simulink model "HANcoder_E407_TTA_Controller_v2"  (R2018b)
settings: Solver=FixedStepDiscrete  StartTime=0.0  StopTime=1  FixedStep=0.01  RelTol=1e-3
PreLoadFcn:
  | librarySetup
  | eval([bdroot,'_startup']) %Calling [modelName]_startup.m
values from neighbouring files (symbols this model uses):
  basic_cycle_duration_bc0 = TM_Reset_Board   + COMP_duration    (= 212)    [HANcoder_E407_TTA_Controller_v3_startup.m]
  basic_cycle_duration_bc1 = TM_Reset_Var_bc1 + COMP_duration    (= 288)    [HANcoder_E407_TTA_Controller_v3_startup.m]
  comm_delay_estimation1 = round(comm_delay_measured1*hardware_granularity/frequency_IRQ)    [HANcoder_E407_TTA_Controller_v3_startup.m]
  comm_delay_estimation2 = round(comm_delay_measured2*hardware_granularity/frequency_IRQ)    [HANcoder_E407_TTA_Controller_v3_startup.m]
  COMM_Period = 40    [HANcoder_E407_TTA_Controller_v3_startup.m]
  COMM_Phase1 = Simulink.Parameter    [HANcoder_E407_TTA_Controller_v3_startup.m]
  COMM_Phase2 = Simulink.Parameter    [HANcoder_E407_TTA_Controller_v3_startup.m]
  COMP_duration = 4    [HANcoder_E407_TTA_Controller_v3_startup.m]
  Controller1_Board = 1    [HANcoder_E407_TTA_Controller_v3_startup.m]
  Controller2_Board = 2    [HANcoder_E407_TTA_Controller_v3_startup.m]
  Controller3_Board = 3    [HANcoder_E407_TTA_Controller_v3_startup.m]
  delta_max = 1    [HANcoder_E407_TTA_Controller_v3_startup.m]
  delta_min = -1    [HANcoder_E407_TTA_Controller_v3_startup.m]
  delta_precision = 6    [HANcoder_E407_TTA_Controller_v3_startup.m]
  e_width = 0.1    [HANcoder_E407_TTA_Controller_v3_startup.m]
  frequency_IRQ = 100    [HANcoder_E407_TTA_Controller_v3_startup.m]
  HANtuneOverride = Simulink.Parameter    [HANcoder_E407_TTA_Controller_v3_startup.m]
  hardware_granularity = 1000000    [HANcoder_E407_TTA_Controller_v3_startup.m]
  I_a = 2.25    [HANcoder_E407_TTA_Controller_v3_startup.m]
  I_f = 2.25    [HANcoder_E407_TTA_Controller_v3_startup.m]
  idle_time_init = basic_cycle_duration_bc0 + basic_cycle_duration_bc1    (= 500)    [HANcoder_E407_TTA_Controller_v3_startup.m]
  Input_Gen_Board = 4    [HANcoder_E407_TTA_Controller_v3_startup.m]
  LA_Clock_Gr = 1    [HANcoder_E407_TTA_Controller_v3_startup.m]
  LA_COMM_Err = 1    [HANcoder_E407_TTA_Controller_v3_startup.m]
  LA_MEX_Flag = 1    [HANcoder_E407_TTA_Controller_v3_startup.m]
  LA_Task_Act = 1    [HANcoder_E407_TTA_Controller_v3_startup.m]
  m_v = 100.0    (= 100)    [HANcoder_E407_TTA_Controller_v3_startup.m]
  Master_Role = 1    [HANcoder_E407_TTA_Controller_v3_startup.m]
  matrix_cycle_duration = basic_cycle_duration_bc0 + basic_cycle_duration_bc1    (= 500)    [HANcoder_E407_TTA_Controller_v3_startup.m]
  matrix_rows = 2    [HANcoder_E407_TTA_Controller_v3_startup.m]
  max_num_msgs_CAN1 = 2^Tx_bit_number-1    (= 7)    [HANcoder_E407_TTA_Controller_v3_startup.m]
  max_num_msgs_CAN2 = max_num_msgs_CAN1    (= 7)    [HANcoder_E407_TTA_Controller_v3_startup.m]
  OutControl1_ID = 23    [HANcoder_E407_TTA_Controller_v3_startup.m]
  OutControl2_ID = 24    [HANcoder_E407_TTA_Controller_v3_startup.m]
  OutEmulator_ID = 25    [HANcoder_E407_TTA_Controller_v3_startup.m]
  R_al = 0.10    (= 0.1)    [HANcoder_E407_TTA_Controller_v3_startup.m]
  R_ar = 0.10    (= 0.1)    [HANcoder_E407_TTA_Controller_v3_startup.m]
  R_fl = 0.10    (= 0.1)    [HANcoder_E407_TTA_Controller_v3_startup.m]
  R_fr = 0.10    (= 0.1)    [HANcoder_E407_TTA_Controller_v3_startup.m]
  SensorValues_ID = 22    [HANcoder_E407_TTA_Controller_v3_startup.m]
  SetValues_ID = 21    [HANcoder_E407_TTA_Controller_v3_startup.m]
  Slave_Role = 2    [HANcoder_E407_TTA_Controller_v3_startup.m]
  speed_k_d = Simulink.Parameter    [HANcoder_E407_TTA_Controller_v3_startup.m]
  speed_k_i = Simulink.Parameter    [HANcoder_E407_TTA_Controller_v3_startup.m]
  speed_k_p = Simulink.Parameter    [HANcoder_E407_TTA_Controller_v3_startup.m]
  speed_max = 10    [HANcoder_E407_TTA_Controller_v3_startup.m]
  speed_min = -10    [HANcoder_E407_TTA_Controller_v3_startup.m]
  speed_precision = 3    [HANcoder_E407_TTA_Controller_v3_startup.m]
  Sync_ID = 1    [HANcoder_E407_TTA_Controller_v3_startup.m]
  tau_max = 5    [HANcoder_E407_TTA_Controller_v3_startup.m]
  tau_min = -5    [HANcoder_E407_TTA_Controller_v3_startup.m]
  tau_range = abs(tau_max) + abs(tau_min)    [HANcoder_E407_TTA_Controller_v3_startup.m]
  theta_max = (speed_max/R_fr)*matrix_cycle_duration*frequency_IRQ/hardware_granularity    (= 5)    [HANcoder_E407_TTA_Controller_v3_startup.m]
  theta_min = (-1)*theta_max    (= -5)    [HANcoder_E407_TTA_Controller_v3_startup.m]
  theta_precision = 7-(fix(log2(theta_max))+1)    [HANcoder_E407_TTA_Controller_v3_startup.m]
  Tl_a = 0.6    [HANcoder_E407_TTA_Controller_v3_startup.m]
  Tl_f = 0.6    [HANcoder_E407_TTA_Controller_v3_startup.m]
  TM_Check_Output_Control1 = TM_COMM_Output_Control1 + COMM_duration    (= 188)    [HANcoder_E407_TTA_Controller_v3_startup.m]
  TM_Check_Output_Control2 = TM_COMM_Output_Control2 + COMM_duration    (= 232)    [HANcoder_E407_TTA_Controller_v3_startup.m]
  TM_Check_Output_Emulator = TM_COMM_Output_Emulator + COMM_duration    (= 280)    [HANcoder_E407_TTA_Controller_v3_startup.m]
  TM_Check_Sensor_Values = TM_COMM_Sensor_Values + COMM_duration    (= 132)    [HANcoder_E407_TTA_Controller_v3_startup.m]
  TM_Check_Set_Values = TM_COMM_Set_Values + COMM_duration    (= 88)    [HANcoder_E407_TTA_Controller_v3_startup.m]
  TM_Check_Sync = TM_COMM_Sync   + COMM_duration    (= 40)    [HANcoder_E407_TTA_Controller_v3_startup.m]
  TM_Check_TOuts = TM_Count_Vote3 + COMP_duration    (= 196)    [HANcoder_E407_TTA_Controller_v3_startup.m]
  TM_Check_Vote1 = TM_COMM_Vote1  + COMM_duration    (= 92)    [HANcoder_E407_TTA_Controller_v3_startup.m]
  TM_Check_Vote2 = TM_COMM_Vote2  + COMM_duration    (= 140)    [HANcoder_E407_TTA_Controller_v3_startup.m]
  TM_Check_Vote3 = TM_COMM_Vote3  + COMM_duration    (= 188)    [HANcoder_E407_TTA_Controller_v3_startup.m]
  TM_COMM_Output_Control1 = TM_Velocity + COMP_duration    (= 148)    [HANcoder_E407_TTA_Controller_v3_startup.m]
  TM_COMM_Output_Control2 = TM_Check_Output_Control1 + COMP_duration    (= 192)    [HANcoder_E407_TTA_Controller_v3_startup.m]
  TM_COMM_Output_Emulator = TM_TMR + COMP_duration    (= 240)    [HANcoder_E407_TTA_Controller_v3_startup.m]
  TM_COMM_Sensor_Values = TM_Check_Set_Values + COMP_duration    (= 92)    [HANcoder_E407_TTA_Controller_v3_startup.m]
  TM_COMM_Set_Values = TM_Update_LT + COMP_duration    (= 48)    [HANcoder_E407_TTA_Controller_v3_startup.m]
  TM_COMM_Sync = basic_cycle_start    (= 0)    [HANcoder_E407_TTA_Controller_v3_startup.m]
  TM_COMM_Vote1 = TM_Vote_Dec    + COMP_duration    (= 52)    [HANcoder_E407_TTA_Controller_v3_startup.m]
  TM_COMM_Vote2 = TM_Count_Vote1 + COMP_duration    (= 100)    [HANcoder_E407_TTA_Controller_v3_startup.m]
  TM_COMM_Vote3 = TM_Count_Vote2 + COMP_duration    (= 148)    [HANcoder_E407_TTA_Controller_v3_startup.m]
  TM_Count_Vote1 = TM_Check_Vote1 + COMP_duration    (= 96)    [HANcoder_E407_TTA_Controller_v3_startup.m]
  TM_Count_Vote2 = TM_Check_Vote2 + COMP_duration    (= 144)    [HANcoder_E407_TTA_Controller_v3_startup.m]
  TM_Count_Vote3 = TM_Check_Vote3 + COMP_duration    (= 192)    [HANcoder_E407_TTA_Controller_v3_startup.m]
  TM_Data_bc0 = TM_COMM_Sync    (= 0)    [HANcoder_E407_TTA_Controller_v3_startup.m]
  TM_Data_bc1 = TM_Data_bc0(1:4)    [HANcoder_E407_TTA_Controller_v3_startup.m]
  TM_New_Master = TM_Check_TOuts + COMP_duration    (= 200)    [HANcoder_E407_TTA_Controller_v3_startup.m]
  TM_Reset_Board = TM_Reset_Var   + COMP_duration    (= 208)    [HANcoder_E407_TTA_Controller_v3_startup.m]
  TM_Reset_Var = TM_New_Master  + COMP_duration    (= 204)    [HANcoder_E407_TTA_Controller_v3_startup.m]
  TM_Reset_Var_bc1 = TM_Check_Output_Emulator + COMP_duration    (= 284)    [HANcoder_E407_TTA_Controller_v3_startup.m]
  TM_Steer = TM_Check_Sensor_Values + COMP_duration    (= 136)    [HANcoder_E407_TTA_Controller_v3_startup.m]
  TM_TMR = TM_Check_Output_Control2 + COMP_duration    (= 236)    [HANcoder_E407_TTA_Controller_v3_startup.m]
  TM_Torque = TM_Steer + COMP_duration    (= 140)    [HANcoder_E407_TTA_Controller_v3_startup.m]
  TM_Type_bc0 = COMM    (= 0)    [HANcoder_E407_TTA_Controller_v3_startup.m]
  TM_Type_bc1 = TM_Type_bc0(1:4)    [HANcoder_E407_TTA_Controller_v3_startup.m]
  TM_Update_LT = TM_Check_Sync  + COMP_duration    (= 44)    [HANcoder_E407_TTA_Controller_v3_startup.m]
  TM_Velocity = TM_Torque + COMP_duration    (= 144)    [HANcoder_E407_TTA_Controller_v3_startup.m]
  TM_Vote_Dec = TM_Update_LT   + COMP_duration    (= 48)    [HANcoder_E407_TTA_Controller_v3_startup.m]
  torque_a_k_d = Simulink.Parameter    [HANcoder_E407_TTA_Controller_v3_startup.m]
  torque_a_k_i = Simulink.Parameter    [HANcoder_E407_TTA_Controller_v3_startup.m]
  torque_a_k_p = Simulink.Parameter    [HANcoder_E407_TTA_Controller_v3_startup.m]
  torque_f_k_d = Simulink.Parameter    [HANcoder_E407_TTA_Controller_v3_startup.m]
  torque_f_k_i = Simulink.Parameter    [HANcoder_E407_TTA_Controller_v3_startup.m]
  torque_f_k_p = Simulink.Parameter    [HANcoder_E407_TTA_Controller_v3_startup.m]
  torque_precision = 4    [HANcoder_E407_TTA_Controller_v3_startup.m]
  Vehicle_Em_Board = 5    [HANcoder_E407_TTA_Controller_v3_startup.m]
  Vote1_ID = 11    [HANcoder_E407_TTA_Controller_v3_startup.m]
  Vote2_ID = 12    [HANcoder_E407_TTA_Controller_v3_startup.m]
  Vote3_ID = 13    [HANcoder_E407_TTA_Controller_v3_startup.m]
undefined symbols (not defined in the file or in its folder): A0, A1, A2, A3, A4, CON2
libraries: hdlsllib x235, HANcoder_STM32_Target x25, simulink x3, simulink_extras x1
(part 2 of 22)

== system HANcoder_E407_TTA_Controller_v2/HANcoder STM32 Target - E407-STM32 algorithm/Global Ticks Increment/CAN2 Send ==
  note: Logic Analyzer - DEBUG
      | Message in transmission!
  note: Function call counter
  note: Log Activation CAN send
  note: DEBUG
  note: Logic Analyzer - DEBUG
  note: Transmission message count
      | Update
  Trigger : TriggerPort  TriggerType=function-call  VariantControl=Variant  PortDimensions=1
  Bus Selector : BusSelector  OutputSignals=Buffer_1,Buffer_2,Buffer_3,Buffer_4,Buffer_5,Buffer_6,Buffer_7,Buffer_8
  CAN send1 : Subsystem  Tag=HANcoder_TARGET_STM32_E407  AncestorBlock=HANcoder_STM32_Target/STM32-E407/CAN/CAN/CAN send  mask(CAN send){canBus=CAN 2, frameType=Standard (11 bit), inputNumber=8, dataType=uint8, byteOrder=off, tsamp=-1}
      mask prompts: canBus "CAN channel"; frameType "Identifier type"; inputNumber "Input ports"; dataType "Input datatype"; byteOrder "Byte order: Checked = MSB first, unchecked = LSB first."; tsamp "Sample time"
      mask help:
      | Function
      | ==========
      | Send a message on the CAN channel.
      |
      | Parameters
      | ==========
      | CAN channel:           The CAN channel to send the message on.
      | Identifier type:         normal or extended ID's
      | Input ports:              The amount of input ports
      | Input datatype:        The datatype of the input ports
      | Byte order:               Select MSB or LSB first
      | Sample time:            -1 or divisible by base sample time [seconds]
      |
      | Input
      | ==========
      | Port 1:                   CAN ID(uint32) in hexadecimal ie: hex2dec('0a')
      | Port 2..9                CAN message data
      mask init:
      | sfcn_can_send_mcb(canBus, frameType, inputNumber, dataType, byteOrder)
      settings: MoveFcn=drawLogos
      mask Help: web('sfcn_can_send.html');
      mask TypeOptions canBus: CAN 1 | CAN 2
      mask TypeOptions frameType: Standard (11 bit) | Extended (29 bit)
      mask TypeOptions dataType: int8 | uint8 | int16 | uint16 | int32 | uint32 | boolean
      mask Display:
      | fprintf('Send on\nCAN %x', canBus);
      | port_label('input', 1, 'ID');patch([140 146 146],[8 14 2],[1 0 0]);patch([148 148 154],[14 2 8],[0 0 0.35]);
  Cast To Double : DataTypeConversion  OutDataTypeStr=double
  Constant : Constant  OutDataTypeStr=boolean
  Constant3 : Constant  OutDataTypeStr=uint32
  Constant8 : Constant  Priority=2
  Data Store Memory1 : DataStoreMemory  DataStoreName=fcn_call_counter  ReadBeforeWriteMsg=warning  WriteAfterWriteMsg=warning  WriteAfterReadMsg=warning  ShowAdditionalParam=off  OutDataTypeStr=uint32
  Data Store Read : DataStoreRead  DataStoreName=fcn_call_counter
  Data Store Read1 : DataStoreRead  DataStoreName=Local_Ticks
  Data Store Read2 : DataStoreRead  DataStoreName=Msg_Tx_CAN2
  Data Store Read3 : DataStoreRead  DataStoreName=TxID_CAN2
  Data Store Read4 : DataStoreRead  Priority=1  DataStoreName=Tx_msg_count_CAN2
  Data Store Write : DataStoreWrite  DataStoreName=fcn_call_counter
  Data Store Write1 : DataStoreWrite  DataStoreName=Toggle_Pin_A0
  Data Store Write2 : DataStoreWrite  Priority=4  DataStoreName=Tx_msg_count_CAN2
  Data Type Conversion{,4..10} (8 alike) : DataTypeConversion  OutDataTypeStr=uint8
  Data Type Conversion1 : DataTypeConversion  OutDataTypeStr=uint32
  Get Free Running Counter1 : HANcoder_STM32_Target/STM32-E407/Timer Outputs/Get Free Running Counter  Tag=HANcoder_TARGET_STM32_E407  moduleID=TIM4 - CON PD - 15 & 16 &n/a & n/a  tsamp=-1
      settings: SourceProductName=HANcoder STM32 Target
  Plus : Sum  Priority=3
  Sum1 : Sum
  Terminator : Terminator
  Terminator4 : Terminator
  Terminator5 : Terminator
  wires:
  Constant/1 -> Data Store Write1/1
  Get Free Running Counter1/1 -> Terminator5/1  "FRC_Activation_CAN2_send"
  Data Store Read1/1 -> Terminator4/1  "Local_Ticks_Activation_CAN2_send"
  Sum1/1 -> Data Store Write/1  "TxCAN2_counter_s"
  Data Store Read/1 -> Sum1/2
  Constant3/1 -> Sum1/1
  Data Type Conversion7/1 -> CAN send1/6(In6)
  Data Type Conversion6/1 -> CAN send1/5(In5)
  Data Type Conversion4/1 -> CAN send1/3(In3)
  Data Type Conversion5/1 -> CAN send1/4(In4)
  Data Type Conversion8/1 -> CAN send1/7(In7)
  Data Type Conversion9/1 -> CAN send1/8(In8)
  Data Type Conversion1/1 -> CAN send1/1(In1)
  Data Type Conversion/1 -> CAN send1/2(In2)
  Data Type Conversion10/1 -> CAN send1/9(In9)
  Data Store Read3/1 -> Data Type Conversion1/1  "TxID_CAN2_s"
  Bus Selector/3 -> Data Type Conversion5/1  "<Buffer_3>"
  Bus Selector/2 -> Data Type Conversion4/1  "<Buffer_2>"
  Bus Selector/6 -> Data Type Conversion8/1  "<Buffer_6>"
  Bus Selector/4 -> Data Type Conversion6/1  "<Buffer_4>"
  Bus Selector/8 -> Data Type Conversion10/1  "<Buffer_8>"
  Data Store Read2/1 -> Bus Selector/1
  Bus Selector/7 -> Data Type Conversion9/1  "<Buffer_7>"
  Bus Selector/5 -> Data Type Conversion7/1  "<Buffer_5>"
  Data Store Read4/1 -> Plus/1
  Plus/1 -> Data Store Write2/1
  Constant8/1 -> Plus/2
  Bus Selector/1 -> Cast To Double/1, Data Type Conversion/1  "<Buffer_1>"
  Cast To Double/1 -> Terminator/1  "Tx_temporal_msg_CAN2"

== system HANcoder_E407_TTA_Controller_v2/HANcoder STM32 Target - E407-STM32 algorithm/Global Ticks Increment/If Action Subsystem ==
  note: CAN ID Init
  Action Port : ActionPort  ActionType=then
  Add : Sum  Inputs=++++
  Constant : Constant
  Constant1 : Constant  Value=2
  Constant2 : Constant  Value=4
  Constant3 : Constant  Value=8
  Digital Input4 : HANcoder_STM32_Target/STM32-E407/Digital Inputs/Digital Input  Tag=HANcoder_TARGET_STM32_E407  pinID=CON3 - D2 - 5V Tolerant  config=Pulldown  tsamp=-1
      settings: SourceProductName=HANcoder STM32 Target
  Digital Input5 : HANcoder_STM32_Target/STM32-E407/Digital Inputs/Digital Input  Tag=HANcoder_TARGET_STM32_E407  pinID=CON3 - D3 - 5V Tolerant  config=Pulldown  tsamp=-1
      settings: SourceProductName=HANcoder STM32 Target
  Digital Input6 : HANcoder_STM32_Target/STM32-E407/Digital Inputs/Digital Input  Tag=HANcoder_TARGET_STM32_E407  pinID=CON3 - D4 - 5V Tolerant  config=Pulldown  tsamp=-1
      settings: SourceProductName=HANcoder STM32 Target
  Digital Input7 : HANcoder_STM32_Target/STM32-E407/Digital Inputs/Digital Input  Tag=HANcoder_TARGET_STM32_E407  pinID=CON3 - D5 - 5V Tolerant  config=Pulldown  tsamp=-1
      settings: SourceProductName=HANcoder STM32 Target
  Multiply{,1..3} (4 alike) : Product
  Out1 : Outport
  wires:
  Constant1/1 -> Multiply1/1
  Add/1 -> Out1/1
  Constant3/1 -> Multiply3/1
  Constant2/1 -> Multiply2/1
  Multiply2/1 -> Add/3
  Digital Input7/1 -> Multiply3/2
  Digital Input5/1 -> Multiply1/2
  Multiply3/1 -> Add/4
  Multiply1/1 -> Add/2
  Digital Input6/1 -> Multiply2/2
  Multiply/1 -> Add/1
  Digital Input4/1 -> Multiply/2
  Constant/1 -> Multiply/1

== system HANcoder_E407_TTA_Controller_v2/HANcoder STM32 Target - E407-STM32 algorithm/Global Ticks Increment/Initialize Clock Schedule ==
  Enable : EnablePort
  Constant : Constant  OutDataTypeStr=uint16
  Constant1 : Constant  Value=3  OutDataTypeStr=uint8
  Constant2 : Constant
  Data Store Write : DataStoreWrite  DataStoreName=init_clock
  Schedule Compare Event : HANcoder_STM32_Target/STM32-E407/Timer Outputs/Schedule Compare Event  Tag=HANcoder_TARGET_STM32_E407  pin=TIM4 - CON PD - 15 - 5V Tolerant  tsamp=-1
      settings: SourceProductName=HANcoder STM32 Target
  wires:
  Constant/1 -> Schedule Compare Event/1
  Constant1/1 -> Schedule Compare Event/2
  Constant2/1 -> Data Store Write/1

== system HANcoder_E407_TTA_Controller_v2/HANcoder STM32 Target - E407-STM32 algorithm/Global Ticks Increment/Local Time generation ==
  note: Reschedule IRQ activation
  Clock_State : Inport
  function : TriggerPort  TriggerType=function-call  VariantControl=Variant
  Chart : Stateflow chart  TreatAsAtomicUnit=on
  Constant : Constant  Value=frequency_IRQ  OutDataTypeStr=uint16
  Constant1 : Constant  Value=3  OutDataTypeStr=uint8
  Constant2 : Constant  OutDataTypeStr=uint16
  Data Store Read : DataStoreRead  DataStoreName=Local_Ticks
  Data Store Read1 : DataStoreRead  DataStoreName=Local_Ticks
  Data Store Write : DataStoreWrite  DataStoreName=Local_Ticks
  Get Last Event Counter : HANcoder_STM32_Target/STM32-E407/Timer Outputs/Get Last Event Counter  Tag=HANcoder_TARGET_STM32_E407  pin=TIM4 - CON PD - 15 - 5V Tolerant  tsamp=-1
      settings: SourceProductName=HANcoder STM32 Target
  Schedule Compare Event1 : HANcoder_STM32_Target/STM32-E407/Timer Outputs/Schedule Compare Event  Tag=HANcoder_TARGET_STM32_E407  pin=TIM4 - CON PD - 15 - 5V Tolerant  tsamp=-1
      settings: SourceProductName=HANcoder STM32 Target
  Sum : Sum
  Sum1 : Sum
  Switch : Switch  Criteria=u2 > Threshold
  activate_CAN_management : Outport
  wires:
  Get Last Event Counter/1 -> Sum/1
  Constant/1 -> Sum/2
  Sum/1 -> Schedule Compare Event1/1
  Constant1/1 -> Schedule Compare Event1/2
  Data Store Read1/1 -> Switch/3
  Data Store Read/1 -> Sum1/1
  Constant2/1 -> Sum1/2
  Clock_State/1 -> Chart/1(Condition), Switch/2
  Switch/1 -> Data Store Write/1  "local_ticks_interrupt"
  Sum1/1 -> Switch/1
  Chart/1(Trigger_Signal()) -> activate_CAN_management/1

== system HANcoder_E407_TTA_Controller_v2/HANcoder STM32 Target - E407-STM32 algorithm/Global Ticks Increment/Measure EXecution time ==
  note: Measured Execution Time
  Trigger : TriggerPort  TriggerType=function-call  VariantControl=Variant
  Constant1 : Constant  Priority=1  Value=LA_MEX_Flag
  DEBUG - Toggle digital pin A3 : Subsystem  Priority=3
  Data Store Memory4 : DataStoreMemory  DataStoreName=A3_Pin_State  ReadBeforeWriteMsg=warning  WriteAfterWriteMsg=warning  WriteAfterReadMsg=warning  ShowAdditionalParam=off  OutDataTypeStr=boolean
  wires:
  Constant1/1 -> DEBUG - Toggle digital pin A3/Enable

== system HANcoder_E407_TTA_Controller_v2/HANcoder STM32 Target - E407-STM32 algorithm/Global Ticks Increment/Output Compare Init ==
  S-Function : S-Function  FunctionName=sfcn_timeout_init  SFunctionDeploymentMode=off  EnableBusSupport=off
  Term1 : Terminator
  wires:
  S-Function/1 -> Term1/1

== system HANcoder_E407_TTA_Controller_v2/HANcoder STM32 Target - E407-STM32 algorithm/Operation Mode/Flip Flop T ==
  T : Inport  OutDataTypeStr=boolean
  Clk : Inport  Port=2  OutDataTypeStr=boolean
  J-K Flip-Flop : simulink_extras/Flip Flops/J-K Flip-Flop  initial_condition=0
      settings: SourceProductName=Simulink
  Terminator : Terminator
  Q : Outport  OutDataTypeStr=boolean
  wires:
  J-K Flip-Flop/2 -> Terminator/1
  T/1 -> J-K Flip-Flop/3, J-K Flip-Flop/1
  J-K Flip-Flop/1 -> Q/1
  Clk/1 -> J-K Flip-Flop/2

== system HANcoder_E407_TTA_Controller_v2/HANcoder STM32 Target - E407-STM32 algorithm/Global Ticks Increment/CAN Management/Basic Cycle Increment ==
  note: Local Time Reset
  note: Basic cycle counter
  Enable : EnablePort
  Add : Sum
  Add1 : Sum  Inputs=+-
  Cast : DataTypeConversion  OutDataTypeStr=uint8
  Constant : Constant  Value=matrix_rows
  Data Store Read4 : DataStoreRead  DataStoreName=basic_cycle_count
  Data Store Read5 : DataStoreRead  DataStoreName=basic_cycle_count
  Data Store Write : DataStoreWrite  DataStoreName=Local_Ticks
  Data Store Write3 : DataStoreWrite  DataStoreName=basic_cycle_count
  Decrement : Constant  OutDataTypeStr=uint8
  Increment : Constant  OutDataTypeStr=uint8
  LessThanOrEqual : RelationalOperator  Operator=<  OutDataTypeStr=boolean  RndMeth=Simplest
  Reset : Constant  Value=0  OutDataTypeStr=uint16
  Switch : Switch  Criteria=u2 > Threshold
  wires:
  Switch/1 -> Data Store Write3/1  "bacic_cycle_s"
  Data Store Read5/1 -> LessThanOrEqual/1
  Add/1 -> Switch/1
  Increment/1 -> Add/2
  Data Store Read4/1 -> Add/1
  LessThanOrEqual/1 -> Switch/2
  Constant/1 -> Add1/1
  Reset/1 -> Cast/1, Data Store Write/1
  Decrement/1 -> Add1/2
  Add1/1 -> LessThanOrEqual/2
  Cast/1 -> Switch/3

== system HANcoder_E407_TTA_Controller_v2/HANcoder STM32 Target - E407-STM32 algorithm/Global Ticks Increment/CAN Management/DEBUG - Toggle digital pin A0 ==
  note: Change pin state
  note: Reset condition
  note: Toggle pin data stored
  Enable : EnablePort
  Constant : Constant  OutDataTypeStr=boolean
  Constant1 : Constant  Value=0  OutDataTypeStr=boolean
  Constant2 : Constant  Value=0  OutDataTypeStr=boolean
  Data Store Read : DataStoreRead  DataStoreName=A0_Pin_State
  Data Store Read1 : DataStoreRead  DataStoreName=A0_Pin_State
  Data Store Write : DataStoreWrite  DataStoreName=Toggle_Pin_A0
  Data Store Write1 : DataStoreWrite  DataStoreName=A0_Pin_State
  Digital Output : HANcoder_STM32_Target/STM32-E407/Digital Outputs/Digital Output  Tag=HANcoder_TARGET_STM32_E407  pinID=CON2 - A0  config=Open drain  tsamp=-1
      settings: SourceProductName=HANcoder STM32 Target
  Switch : Switch  Criteria=u2 > Threshold
  wires:
  Switch/1 -> Data Store Write1/1
  Data Store Read/1 -> Switch/2
  Constant/1 -> Switch/3
  Constant1/1 -> Switch/1
  Constant2/1 -> Data Store Write/1
  Data Store Read1/1 -> Digital Output/1

== system HANcoder_E407_TTA_Controller_v2/HANcoder STM32 Target - E407-STM32 algorithm/Global Ticks Increment/CAN Management/DEBUG - Toggle digital pin A1 ==
  note: Toggle pin data stored
  note: Reset condition
  note: Change pin state
  Enable : EnablePort
  Constant : Constant  OutDataTypeStr=boolean
  Constant1 : Constant  Value=0  OutDataTypeStr=boolean
  Constant2 : Constant  Value=0  OutDataTypeStr=boolean
  Data Store Read : DataStoreRead  DataStoreName=A1_Pin_State
  Data Store Read1 : DataStoreRead  DataStoreName=A1_Pin_State
  Data Store Write : DataStoreWrite  DataStoreName=Toggle_Pin_A1
  Data Store Write1 : DataStoreWrite  DataStoreName=A1_Pin_State
  Digital Output : HANcoder_STM32_Target/STM32-E407/Digital Outputs/Digital Output  Tag=HANcoder_TARGET_STM32_E407  pinID=CON2 - A1  config=Open drain  tsamp=-1
      settings: SourceProductName=HANcoder STM32 Target
  Switch : Switch  Criteria=u2 > Threshold
  wires:
  Data Store Read1/1 -> Digital Output/1
  Constant2/1 -> Data Store Write/1
  Constant1/1 -> Switch/1
  Constant/1 -> Switch/3
  Data Store Read/1 -> Switch/2
  Switch/1 -> Data Store Write1/1

== system HANcoder_E407_TTA_Controller_v2/HANcoder STM32 Target - E407-STM32 algorithm/Global Ticks Increment/CAN Management/DEBUG - Toggle digital pin A2 ==
  note: Toggle pin data stored
  note: Change pin state
  Enable : EnablePort
  Constant : Constant  OutDataTypeStr=boolean
  Constant1 : Constant  Value=0  OutDataTypeStr=boolean
  Data Store Read : DataStoreRead  DataStoreName=A2_Pin_State
  Data Store Read1 : DataStoreRead  DataStoreName=A2_Pin_State
  Data Store Write1 : DataStoreWrite  DataStoreName=A2_Pin_State
  Digital Output : HANcoder_STM32_Target/STM32-E407/Digital Outputs/Digital Output  Tag=HANcoder_TARGET_STM32_E407  pinID=CON2 - A2  config=Open drain  tsamp=-1
      settings: SourceProductName=HANcoder STM32 Target
  Switch : Switch  Criteria=u2 > Threshold
  wires:
  Data Store Read1/1 -> Digital Output/1
  Constant1/1 -> Switch/1
  Constant/1 -> Switch/3
  Data Store Read/1 -> Switch/2
  Switch/1 -> Data Store Write1/1

== system HANcoder_E407_TTA_Controller_v2/HANcoder STM32 Target - E407-STM32 algorithm/Global Ticks Increment/CAN Management/DEBUG - Toggle digital pin A4 ==
  note: Toggle pin data stored
  note: Change pin state
  Enable : EnablePort
  Constant : Constant  OutDataTypeStr=boolean
  Constant1 : Constant  Value=0  OutDataTypeStr=boolean
  Data Store Read : DataStoreRead  DataStoreName=A4_Pin_State
  Data Store Read1 : DataStoreRead  DataStoreName=A4_Pin_State
  Data Store Write1 : DataStoreWrite  DataStoreName=A4_Pin_State
  Digital Output : HANcoder_STM32_Target/STM32-E407/Digital Outputs/Digital Output  Tag=HANcoder_TARGET_STM32_E407  pinID=CON2 - A4  config=Open drain  tsamp=-1
      settings: SourceProductName=HANcoder STM32 Target
  Switch : Switch  Criteria=u2 > Threshold
  wires:
  Data Store Read1/1 -> Digital Output/1
  Constant1/1 -> Switch/1
  Constant/1 -> Switch/3
  Data Store Read/1 -> Switch/2
  Switch/1 -> Data Store Write1/1

== system HANcoder_E407_TTA_Controller_v2/HANcoder STM32 Target - E407-STM32 algorithm/Global Ticks Increment/CAN Management/Initialization ==
  Enable : EnablePort  PropagateVarSize=During execution
  AND : Logic  IconShape=distinctive  AllPortsSameDT=off  OutDataTypeStr=boolean
  Board nr1 : Constant
  Constant : Constant  Value=idle_time_init
  Data Store Memory : DataStoreMemory  DataStoreName=Initialization_Timeout  ReadBeforeWriteMsg=warning  WriteAfterWriteMsg=warning  WriteAfterReadMsg=warning  ShowAdditionalParam=off  OutDataTypeStr=boolean
  Data Store Memory1 : DataStoreMemory  DataStoreName=Delay_Counter  ReadBeforeWriteMsg=warning  WriteAfterWriteMsg=warning  WriteAfterReadMsg=warning  ShowAdditionalParam=off  OutDataTypeStr=double
  Data Store Read : DataStoreRead  DataStoreName=New_Msg_Ready_CAN1
  Data Store Read1 : DataStoreRead  DataStoreName=Initialization_Timeout
  Data Store Read2 : DataStoreRead  DataStoreName=New_Msg_Ready_CAN2
  Data Store Read4 : DataStoreRead  DataStoreName=Board_ID
  Data Store Write : DataStoreWrite  DataStoreName=Initialization_Timeout
  Data Store Write1 : DataStoreWrite  DataStoreName=Initialization_flag
  Delay : Subsystem
  Equal : RelationalOperator  Operator===  OutDataTypeStr=boolean  RndMeth=Simplest
  NOT : Logic  Operator=NOT  IconShape=distinctive  AllPortsSameDT=off  OutDataTypeStr=boolean
  OR : Logic  Operator=OR  IconShape=distinctive  AllPortsSameDT=off  OutDataTypeStr=boolean
  OR1 : Logic  Operator=OR  IconShape=distinctive  AllPortsSameDT=off  OutDataTypeStr=boolean
  RoleID and Global Time init : Subsystem  TreatAsAtomicUnit=on
  wires:
  Delay/1(Output) -> Data Store Write/1
  Constant/1 -> Delay/1(Input)
  NOT/1 -> Data Store Write1/1
  RoleID and Global Time init/1(Finish Initialization) -> NOT/1
  OR/1 -> RoleID and Global Time init/Enable
  Data Store Read1/1 -> AND/2, RoleID and Global Time init/1(Timeout Initialization)
  OR1/1 -> OR/2, RoleID and Global Time init/2(Reference message received)
  Data Store Read4/1 -> Equal/1
  Board nr1/1 -> Equal/2
  Equal/1 -> AND/1
  AND/1 -> OR/1
  Data Store Read/1 -> OR1/1
  Data Store Read2/1 -> OR1/2

== system HANcoder_E407_TTA_Controller_v2/HANcoder STM32 Target - E407-STM32 algorithm/Global Ticks Increment/CAN Management/LT_Update Desync_Positive ==
  note: Local Time Update with Positive Desync
      | This subsystem is only activated if we have to update
      | the local time with a positive desync. This is activated
      | at the end of the current Computational Task, so the
      | Local Time is updated until the tick before the next
      | Computational Task in the basic cycle. This way we
      | avoid missing tasks, as would happened when updating
      | the Local Time too quickly into the future.
  note: WARNING
      | TM_Type is currently defined as
      | COMM type 0
      | COMP type 1
  note: Constants bc0
  note: constants are defined in the _startup file
  note: Constants bc1
  Local Time : Inport
  Bacic_Cycle : Inport  Port=2
  Enable : EnablePort  PropagateVarSize=During execution
  Bus Selector : BusSelector  OutputSignals=signal1,signal2
  Bus Creator : BusCreator  Inputs=2
  Bus Creator1 : BusCreator  Inputs=2
  Constant : Constant  Value=TM_Data_bc0
  Constant1 : Constant  Value=TM_Type_bc0
  Constant2 : Constant  Value=COMM_Phase1
  Constant3 : Constant  Value=COMM_Phase2
  Constant4 : Constant  Value=TM_Data_bc1
  Constant5 : Constant  Value=TM_Type_bc1
  Constant8 : Constant  Value=0
  Equal : RelationalOperator  Operator===  OutDataTypeStr=boolean  RndMeth=Simplest
  Local Time Update with Positive Desync : Subsystem  TreatAsAtomicUnit=on
  MATLAB Function : MATLAB Function  TreatAsAtomicUnit=on
  Switch : Switch  Criteria=u2 > Threshold  AllowDiffInputSizes=on
  wires:
  MATLAB Function/1(result_time) -> Local Time Update with Positive Desync/1(Ticks until next COMP)
  Local Time/1 -> MATLAB Function/1(local_time)
  Constant8/1 -> Equal/2
  Bacic_Cycle/1 -> Equal/1
  Equal/1 -> Switch/2
  Constant/1 -> Bus Creator/1
  Constant1/1 -> Bus Creator/2
  Bus Creator/1 -> Switch/1
  Constant4/1 -> Bus Creator1/1
  Constant5/1 -> Bus Creator1/2
  Bus Creator1/1 -> Switch/3
  Switch/1 -> Bus Selector/1
  Bus Selector/1 -> MATLAB Function/2(TM_data)  "<signal1>"
  Bus Selector/2 -> MATLAB Function/3(TM_type)  "<signal2>"
  Constant3/1 -> MATLAB Function/5(phase2)
  Constant2/1 -> MATLAB Function/4(phase1)

== system HANcoder_E407_TTA_Controller_v2/HANcoder STM32 Target - E407-STM32 algorithm/Global Ticks Increment/CAN Management/Matrix Cycle Manager ==
  note: Controller boards condition
  note: Output Send_Message
      | Send: 1
      | Do not send: 0
  note: Output Receive_Message
      | Receive: 1
      | Do not receive: 0
  note: Output Receive_Message
      | Receive: 1
      | Do not receive: 0
  note: Output Send_Message
      | Send: 1
      | Do not send: 0
  Enable : EnablePort  PropagateVarSize=During execution
  Bus Selector : BusSelector  OutputSignals=signal1,signal2,signal3,signal4
  Bus Creator : BusCreator  Inputs=4
  Constant : Constant  Value=Controller1_Board
  Constant1 : Constant  Value=Controller2_Board
  Constant2 : Constant  Value=Controller3_Board
  Data Store Read : DataStoreRead  DataStoreName=Board_ID
  Data Store Read10 : DataStoreRead  DataStoreName=basic_cycle_count
  Equal : RelationalOperator  Operator===  OutDataTypeStr=boolean  RndMeth=Simplest
  Equal1 : RelationalOperator  Operator===  OutDataTypeStr=boolean  RndMeth=Simplest
  Equal2 : RelationalOperator  Operator===  OutDataTypeStr=boolean  RndMeth=Simplest
  OR : Logic  Operator=OR  Inputs=3  IconShape=distinctive  AllPortsSameDT=off  OutDataTypeStr=boolean
  Subsystem : Subsystem
  Send_Message_CAN1 : Outport  OutputWhenDisabled=reset  InitialOutput=0
  Send_Message_CAN2 : Outport  Port=2  OutputWhenDisabled=reset  InitialOutput=0
  Receive_Message_CAN1 : Outport  Port=3  OutputWhenDisabled=reset  InitialOutput=0
  Receive_Message_CAN2 : Outport  Port=4  OutputWhenDisabled=reset  InitialOutput=0
  wires:
  Data Store Read10/1 -> Subsystem/1(basic_cycle)
  Constant/1 -> Equal/2
  Constant1/1 -> Equal1/2
  Constant2/1 -> Equal2/2
  Equal/1 -> OR/1
  Equal1/1 -> OR/2
  Equal2/1 -> OR/3
  Data Store Read/1 -> Equal2/1, Equal1/1, Equal/1
  OR/1 -> Subsystem/Enable
  Subsystem/1(Send_CAN1) -> Bus Creator/1
  Subsystem/2(Send_CAN2) -> Bus Creator/2
  Subsystem/3(Receive_CAN1) -> Bus Creator/3
  Subsystem/4(Receive_CAN2) -> Bus Creator/4
  ? -> ?
  Bus Creator/1 -> Bus Selector/1
  Bus Selector/4 -> Receive_Message_CAN2/1  "<signal4>"
  Bus Selector/3 -> Receive_Message_CAN1/1  "<signal3>"
  Bus Selector/2 -> Send_Message_CAN2/1  "<signal2>"
  Bus Selector/1 -> Send_Message_CAN1/1  "<signal1>"

== system HANcoder_E407_TTA_Controller_v2/HANcoder STM32 Target - E407-STM32 algorithm/Global Ticks Increment/CAN1 Recieve/Buffer ready ==
  note: CAN_Rx - Buffer
      | ready for new message
  note: Logic Analyzer - DEBUG
      | Rx Buffer Ready
  Enable : EnablePort
  Data Store Write : DataStoreWrite  DataStoreName=Rx_State_CAN1
  Data Store Write1 : DataStoreWrite  DataStoreName=Toggle_Pin_A0
  New_Msg : Constant  Value=2  OutDataTypeStr=uint8
  SET : Constant  OutDataTypeStr=boolean
  wires:
  New_Msg/1 -> Data Store Write/1
  SET/1 -> Data Store Write1/1

== system HANcoder_E407_TTA_Controller_v2/HANcoder STM32 Target - E407-STM32 algorithm/Global Ticks Increment/CAN1 Recieve/Prepare buffer ==
  note: Start preparing the buffer
  note: Logic Analyzer - DEBUG
      | Preparing Rx buffer
  Enable : EnablePort
  Constant1 : Constant  OutDataTypeStr=uint8
  Data Store Write : DataStoreWrite  DataStoreName=Rx_State_CAN1
  Data Store Write1 : DataStoreWrite  DataStoreName=Toggle_Pin_A0
  SET : Constant  OutDataTypeStr=boolean
  wires:
  Constant1/1 -> Data Store Write/1
  SET/1 -> Data Store Write1/1

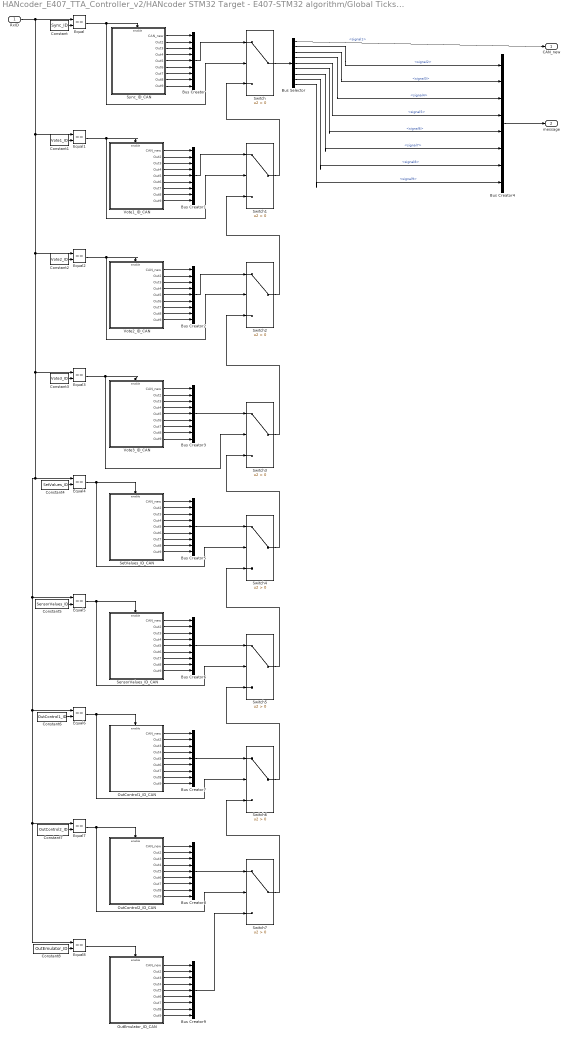
== system HANcoder_E407_TTA_Controller_v2/HANcoder STM32 Target - E407-STM32 algorithm/Global Ticks Increment/CAN1 Recieve/RxID_CAN ==
  RxID : Inport
  Bus Creator4 : BusCreator  Inputs=8
  Bus Selector : BusSelector  OutputSignals=signal1,signal2,signal3,signal4,signal5,signal6,signal7,signal8,signal9
  Bus Creator{,1..3,5..9} (9 alike) : BusCreator  Inputs=9
  Constant : Constant  Value=Sync_ID
  Constant1 : Constant  Value=Vote1_ID
  Constant2 : Constant  Value=Vote2_ID
  Constant3 : Constant  Value=Vote3_ID
  Constant4 : Constant  Value=SetValues_ID
  Constant5 : Constant  Value=SensorValues_ID
  Constant6 : Constant  Value=OutControl1_ID
  Constant7 : Constant  Value=OutControl2_ID
  Constant8 : Constant  Value=OutEmulator_ID
  Equal{,1..8} (9 alike) : RelationalOperator  Operator===  OutDataTypeStr=boolean  RndMeth=Simplest
  OutControl1_ID_CAN : Subsystem
  OutControl2_ID_CAN : Subsystem
  OutEmulator_ID_CAN : Subsystem
  SensorValues_ID_CAN : Subsystem
  SetValues_ID_CAN : Subsystem
  Switch{,1..7} (8 alike) : Switch  Criteria=u2 > Threshold
  Sync_ID_CAN : Subsystem
  Vote1_ID_CAN : Subsystem
  Vote2_ID_CAN : Subsystem
  Vote3_ID_CAN : Subsystem
  CAN_new : Outport
  message : Outport  Port=2
  wires:
  Constant/1 -> Equal/2
  Equal/1 -> Sync_ID_CAN/Enable, Switch/2
  Constant1/1 -> Equal1/2
  Constant2/1 -> Equal2/2
  Constant3/1 -> Equal3/2
  Equal1/1 -> Vote1_ID_CAN/Enable, Switch1/2
  Equal2/1 -> Vote2_ID_CAN/Enable, Switch2/2
  Equal3/1 -> Vote3_ID_CAN/Enable, Switch3/2
  Sync_ID_CAN/1(CAN_new) -> Bus Creator/1
  Sync_ID_CAN/2(Out2) -> Bus Creator/2
  Sync_ID_CAN/3(Out3) -> Bus Creator/3
  Sync_ID_CAN/4(Out4) -> Bus Creator/4
  Sync_ID_CAN/5(Out5) -> Bus Creator/5
  Sync_ID_CAN/6(Out6) -> Bus Creator/6
  Sync_ID_CAN/7(Out7) -> Bus Creator/7
  Sync_ID_CAN/8(Out8) -> Bus Creator/8
  Sync_ID_CAN/9(Out9) -> Bus Creator/9
  Bus Creator/1 -> Switch/1
  Vote1_ID_CAN/1(CAN_new) -> Bus Creator1/1
  Vote1_ID_CAN/2(Out2) -> Bus Creator1/2
  Vote1_ID_CAN/3(Out3) -> Bus Creator1/3
  Vote1_ID_CAN/4(Out4) -> Bus Creator1/4
  Vote1_ID_CAN/5(Out5) -> Bus Creator1/5
  Vote1_ID_CAN/6(Out6) -> Bus Creator1/6
  Vote1_ID_CAN/7(Out7) -> Bus Creator1/7
  Vote1_ID_CAN/8(Out8) -> Bus Creator1/8
  Vote1_ID_CAN/9(Out9) -> Bus Creator1/9
  Bus Creator1/1 -> Switch1/1
  Vote2_ID_CAN/1(CAN_new) -> Bus Creator2/1
  Vote2_ID_CAN/2(Out2) -> Bus Creator2/2
  Vote2_ID_CAN/3(Out3) -> Bus Creator2/3
  Vote2_ID_CAN/4(Out4) -> Bus Creator2/4
  Vote2_ID_CAN/6(Out6) -> Bus Creator2/6
  Vote2_ID_CAN/5(Out5) -> Bus Creator2/5
  Vote2_ID_CAN/7(Out7) -> Bus Creator2/7
  Vote2_ID_CAN/8(Out8) -> Bus Creator2/8
  Vote2_ID_CAN/9(Out9) -> Bus Creator2/9
  Bus Creator2/1 -> Switch2/1
  Vote3_ID_CAN/1(CAN_new) -> Bus Creator3/1
  Vote3_ID_CAN/2(Out2) -> Bus Creator3/2
  Vote3_ID_CAN/3(Out3) -> Bus Creator3/3
  Vote3_ID_CAN/4(Out4) -> Bus Creator3/4
  Vote3_ID_CAN/5(Out5) -> Bus Creator3/5
  Vote3_ID_CAN/6(Out6) -> Bus Creator3/6
  Vote3_ID_CAN/7(Out7) -> Bus Creator3/7
  Vote3_ID_CAN/8(Out8) -> Bus Creator3/8
  Vote3_ID_CAN/9(Out9) -> Bus Creator3/9
  Bus Creator3/1 -> Switch3/1
  Switch1/1 -> Switch/3
  Switch2/1 -> Switch1/3
  Switch/1 -> Bus Selector/1
  Bus Selector/1 -> CAN_new/1  "<signal1>"
  Bus Creator4/1 -> message/1
  Bus Selector/2 -> Bus Creator4/1  "<signal2>"
  Bus Selector/6 -> Bus Creator4/5  "<signal6>"
  Bus Selector/7 -> Bus Creator4/6  "<signal7>"
  Bus Selector/8 -> Bus Creator4/7  "<signal8>"
  Bus Selector/9 -> Bus Creator4/8  "<signal9>"
  Bus Selector/3 -> Bus Creator4/2  "<signal3>"
  Bus Selector/4 -> Bus Creator4/3  "<signal4>"
  Bus Selector/5 -> Bus Creator4/4  "<signal5>"
  Switch3/1 -> Switch2/3
  Switch4/1 -> Switch3/3
  Switch5/1 -> Switch4/3
  SetValues_ID_CAN/9(Out9) -> Bus Creator5/9
  SetValues_ID_CAN/8(Out8) -> Bus Creator5/8
  SetValues_ID_CAN/7(Out7) -> Bus Creator5/7
  SetValues_ID_CAN/6(Out6) -> Bus Creator5/6
  SetValues_ID_CAN/5(Out5) -> Bus Creator5/5
  SetValues_ID_CAN/2(Out2) -> Bus Creator5/2
  SetValues_ID_CAN/1(CAN_new) -> Bus Creator5/1
  SetValues_ID_CAN/3(Out3) -> Bus Creator5/3
  SetValues_ID_CAN/4(Out4) -> Bus Creator5/4
  Bus Creator5/1 -> Switch4/1
  Constant4/1 -> Equal4/2
  Equal4/1 -> SetValues_ID_CAN/Enable, Switch4/2
  Equal5/1 -> Switch5/2, SensorValues_ID_CAN/Enable
  Constant5/1 -> Equal5/2
  Bus Creator6/1 -> Switch5/1
  SensorValues_ID_CAN/4(Out4) -> Bus Creator6/4
  SensorValues_ID_CAN/3(Out3) -> Bus Creator6/3
  SensorValues_ID_CAN/1(CAN_new) -> Bus Creator6/1
  SensorValues_ID_CAN/2(Out2) -> Bus Creator6/2
  SensorValues_ID_CAN/5(Out5) -> Bus Creator6/5
  SensorValues_ID_CAN/6(Out6) -> Bus Creator6/6
  SensorValues_ID_CAN/7(Out7) -> Bus Creator6/7
  SensorValues_ID_CAN/8(Out8) -> Bus Creator6/8
  SensorValues_ID_CAN/9(Out9) -> Bus Creator6/9
  OutControl1_ID_CAN/9(Out9) -> Bus Creator7/9
  OutControl1_ID_CAN/8(Out8) -> Bus Creator7/8
  OutControl1_ID_CAN/7(Out7) -> Bus Creator7/7
  OutControl1_ID_CAN/6(Out6) -> Bus Creator7/6
  OutControl1_ID_CAN/5(Out5) -> Bus Creator7/5
  OutControl1_ID_CAN/2(Out2) -> Bus Creator7/2
  OutControl1_ID_CAN/1(CAN_new) -> Bus Creator7/1
  OutControl1_ID_CAN/3(Out3) -> Bus Creator7/3
  OutControl1_ID_CAN/4(Out4) -> Bus Creator7/4
  Constant6/1 -> Equal6/2
  Equal6/1 -> Switch6/2, OutControl1_ID_CAN/Enable
  Bus Creator7/1 -> Switch6/1
  Bus Creator8/1 -> Switch7/1
  Equal7/1 -> Switch7/2, OutControl2_ID_CAN/Enable
  Constant7/1 -> Equal7/2
  OutControl2_ID_CAN/4(Out4) -> Bus Creator8/4
  OutControl2_ID_CAN/3(Out3) -> Bus Creator8/3
  OutControl2_ID_CAN/1(CAN_new) -> Bus Creator8/1
  OutControl2_ID_CAN/2(Out2) -> Bus Creator8/2
  OutControl2_ID_CAN/5(Out5) -> Bus Creator8/5
  OutControl2_ID_CAN/6(Out6) -> Bus Creator8/6
  OutControl2_ID_CAN/7(Out7) -> Bus Creator8/7
  OutControl2_ID_CAN/8(Out8) -> Bus Creator8/8
  OutControl2_ID_CAN/9(Out9) -> Bus Creator8/9
  OutEmulator_ID_CAN/9(Out9) -> Bus Creator9/9
  OutEmulator_ID_CAN/8(Out8) -> Bus Creator9/8
  OutEmulator_ID_CAN/7(Out7) -> Bus Creator9/7
  OutEmulator_ID_CAN/6(Out6) -> Bus Creator9/6
  OutEmulator_ID_CAN/5(Out5) -> Bus Creator9/5
  OutEmulator_ID_CAN/2(Out2) -> Bus Creator9/2
  OutEmulator_ID_CAN/1(CAN_new) -> Bus Creator9/1
  OutEmulator_ID_CAN/3(Out3) -> Bus Creator9/3
  OutEmulator_ID_CAN/4(Out4) -> Bus Creator9/4
  Constant8/1 -> Equal8/2
  RxID/1 -> Equal2/1, Equal6/1, Equal7/1, Equal8/1, Equal5/1, Equal4/1, Equal3/1, Equal1/1, Equal/1
  Equal8/1 -> OutEmulator_ID_CAN/Enable
  Bus Creator9/1 -> Switch7/3
  Switch7/1 -> Switch6/3
  Switch6/1 -> Switch5/3

== system HANcoder_E407_TTA_Controller_v2/HANcoder STM32 Target - E407-STM32 algorithm/Global Ticks Increment/CAN1 Recieve/Update message buffers ==
  note: Local time when the
      | message is received
  note: Received message
      | ready for processing
  note: CAN_Rx stop listening
  note: Logic Analyzer - DEBUG
      | Message received!
  message : Inport  OutDataTypeStr=Bus: msg_buffer_type
  Enable : EnablePort
  Bus Selector : BusSelector  OutputSignals=signal2,signal3,signal4,signal5,signal6,signal7,signal8,signal9
  Cast To Double : DataTypeConversion  OutDataTypeStr=double
  Data Store Write : DataStoreWrite  DataStoreName=Toggle_Pin_A0
  Data Store Write1 : DataStoreWrite  DataStoreName=Msg_Rx_CAN1  DataStoreElements=Msg_Rx_CAN1.Buffer_1#Msg_Rx_CAN1.Buffer_2#Msg_Rx_CAN1.Buffer_3#Msg_Rx_CAN1.Buffer_4#Msg_Rx_CAN1.Buffer_5#Msg_Rx_CAN1.Buffer_6#Msg_Rx_CAN1.Buffer_7#Msg_Rx_CAN1.Buffer_8
  Data Store Write2 : DataStoreWrite  DataStoreName=New_Msg_Ready_CAN1
  Data Store Write5 : DataStoreWrite  DataStoreName=Rx_State_CAN1
  Data Store Write6 : DataStoreWrite  DataStoreName=Msg_Rx_Ticks_CAN1
  Idle_State : Constant  Value=3  OutDataTypeStr=uint8
  Local_Time : DataStoreRead  DataStoreName=Local_Ticks
  SET : Constant  OutDataTypeStr=boolean
  Terminator : Terminator
  wires:
  Idle_State/1 -> Data Store Write5/1
  SET/1 -> Data Store Write/1, Data Store Write2/1
  Local_Time/1 -> Data Store Write6/1  "Rx_msg_ticks_CAN1"
  message/1 -> Bus Selector/1
  Bus Selector/1 -> Cast To Double/1, Data Store Write1/1  "<signal2>"
  Bus Selector/2 -> Data Store Write1/2  "<signal3>"
  Bus Selector/3 -> Data Store Write1/3  "<signal4>"
  Bus Selector/4 -> Data Store Write1/4  "<signal5>"
  Bus Selector/5 -> Data Store Write1/5  "<signal6>"
  Bus Selector/6 -> Data Store Write1/6  "<signal7>"
  Bus Selector/7 -> Data Store Write1/7  "<signal8>"
  Bus Selector/8 -> Data Store Write1/8  "<signal9>"
  Cast To Double/1 -> Terminator/1  "Rx_temporal_msg_CAN1"

== system HANcoder_E407_TTA_Controller_v2/HANcoder STM32 Target - E407-STM32 algorithm/Global Ticks Increment/CAN1 Send/CAN send ==
  In1 : Inport
  In2 : Inport  Port=2
  In3 : Inport  Port=3
  In4 : Inport  Port=4
  In5 : Inport  Port=5
  In6 : Inport  Port=6
  In7 : Inport  Port=7
  In8 : Inport  Port=8
  In9 : Inport  Port=9
  S-Function : M-S-Function  FunctionName=sfcn_can_send  Parameters=tsamp, canBus, frameType, inputNumber, dataType, byteOrder
  wires:
  In1/1 -> S-Function/1
  In2/1 -> S-Function/2
  In3/1 -> S-Function/3
  In4/1 -> S-Function/4
  In5/1 -> S-Function/5
  In6/1 -> S-Function/6
  In7/1 -> S-Function/7
  In8/1 -> S-Function/8
  In9/1 -> S-Function/9

== system HANcoder_E407_TTA_Controller_v2/HANcoder STM32 Target - E407-STM32 algorithm/Global Ticks Increment/CAN2 Recieve/Buffer ready ==
  note: Logic Analyzer - DEBUG
      | Rx Buffer Ready
  note: CAN_Rx - Buffer
      | ready for new message
  Enable : EnablePort
  Data Store Write : DataStoreWrite  DataStoreName=Rx_State_CAN2
  Data Store Write1 : DataStoreWrite  DataStoreName=Toggle_Pin_A0
  New_Msg : Constant  Value=2  OutDataTypeStr=uint8
  SET : Constant  OutDataTypeStr=boolean
  wires:
  SET/1 -> Data Store Write1/1
  New_Msg/1 -> Data Store Write/1

== system HANcoder_E407_TTA_Controller_v2/HANcoder STM32 Target - E407-STM32 algorithm/Global Ticks Increment/CAN2 Recieve/Prepare buffer ==
  note: Logic Analyzer - DEBUG
      | Preparing Rx buffer
  note: Start preparing the buffer
  Enable : EnablePort
  Constant1 : Constant  OutDataTypeStr=uint8
  Data Store Write : DataStoreWrite  DataStoreName=Rx_State_CAN2
  Data Store Write1 : DataStoreWrite  DataStoreName=Toggle_Pin_A0
  SET : Constant  OutDataTypeStr=boolean
  wires:
  SET/1 -> Data Store Write1/1
  Constant1/1 -> Data Store Write/1
